simulink model "matlabmodel"  (R2021a)
settings: Solver=VariableStepAuto  StartTime=0.0  StopTime=1  RelTol=1e-3
libraries: spsMosfetLib x8, spsDCVoltageSourceLib x2, spsCurrentMeasurementLib x1, spsSeriesRLCBranchLib x1, spsVoltageMeasurementLib x1, spspowerguiLib x1
settings Model: Creator=welcome  LastModifiedBy=SANJAY

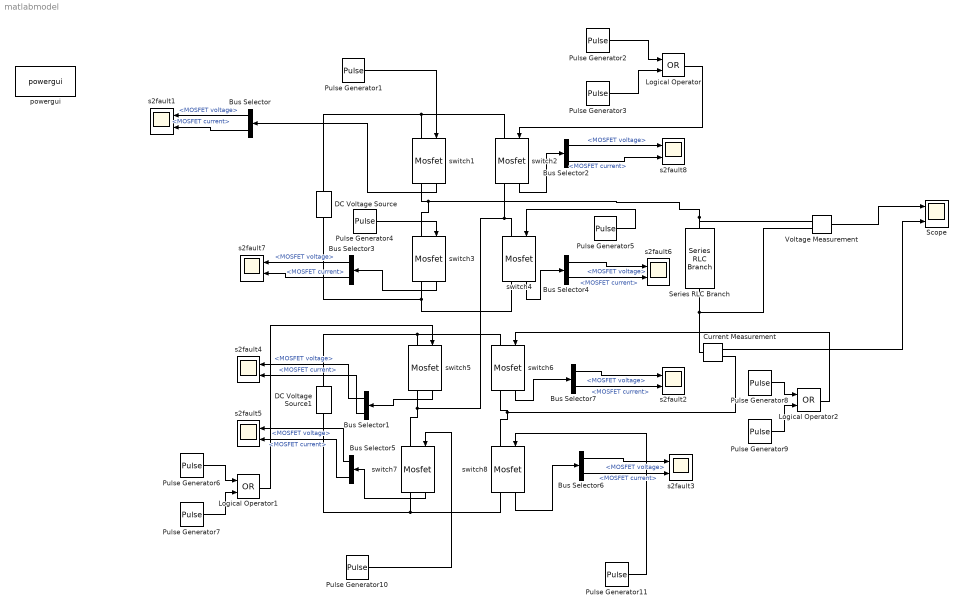
== system matlabmodel ==
  Bus Selector{,1..7} (8 alike) : BusSelector  OutputSignals=MOSFET voltage,MOSFET current
  Current Measurement : spsCurrentMeasurementLib/Current Measurement  PhasorSimulation=off  OutputType=Complex  PSBequivalent=0
  DC Voltage Source : spsDCVoltageSourceLib/DC Voltage Source  Amplitude=100  Measurements=None
  DC Voltage Source1 : spsDCVoltageSourceLib/DC Voltage Source  Amplitude=100  Measurements=None
  Logical Operator : Logic  Operator=OR  AllPortsSameDT=off  OutDataTypeStr=boolean
  Logical Operator1 : Logic  Operator=OR  AllPortsSameDT=off  OutDataTypeStr=boolean
  Logical Operator2 : Logic  Operator=OR  AllPortsSameDT=off  OutDataTypeStr=boolean
  Pulse Generator1 : DiscretePulseGenerator  PulseType=Time based  Period=0.02  PulseWidth=(5/8)*100  PhaseDelay=(0.02/8)*0
  Pulse Generator10 : DiscretePulseGenerator  PulseType=Time based  Period=0.02  PulseWidth=(1/8)*100  PhaseDelay=(0.02/8)*6
  Pulse Generator11 : DiscretePulseGenerator  PulseType=Time based  Period=0.02  PulseWidth=(1/8)*100  PhaseDelay=(0.02/8)*2
  Pulse Generator2 : DiscretePulseGenerator  PulseType=Time based  Period=0.02  PulseWidth=(1/8)*100  PhaseDelay=(0.02/8)*0
  Pulse Generator3 : DiscretePulseGenerator  PulseType=Time based  Period=0.02  PulseWidth=(4/8)*100  PhaseDelay=(0.02/8)*4
  Pulse Generator4 : DiscretePulseGenerator  PulseType=Time based  Period=0.02  PulseWidth=(3/8)*100  PhaseDelay=(0.02/8)*5
  Pulse Generator5 : DiscretePulseGenerator  PulseType=Time based  Period=0.02  PulseWidth=(3/8)*100  PhaseDelay=(0.02/8)*1
  Pulse Generator6 : DiscretePulseGenerator  PulseType=Time based  Period=0.02  PulseWidth=(6/8)*100  PhaseDelay=(0.02/8)*0
  Pulse Generator7 : DiscretePulseGenerator  PulseType=Time based  Period=0.02  PulseWidth=(1/8)*100  PhaseDelay=(0.02/8)*7
  Pulse Generator8 : DiscretePulseGenerator  PulseType=Time based  Period=0.02  PulseWidth=(2/8)*100  PhaseDelay=(0.02/8)*0
  Pulse Generator9 : DiscretePulseGenerator  PulseType=Time based  Period=0.02  PulseWidth=(5/8)*100  PhaseDelay=(0.02/8)*3
  Scope : Scope  NumInputPorts=2
  Series RLC Branch : spsSeriesRLCBranchLib/Series RLC Branch  LConnTagsString=__new0  RConnTagsString=__new0  BranchType=R  Resistance=100  Inductance=1e-3  SetiL0=off  InitialCurrent=0  Capacitance=1e-6  Setx0=off  InitialVoltage=0  Measurements=None
  Voltage Measurement : spsVoltageMeasurementLib/Voltage Measurement  PhasorSimulation=off  OutputType=Complex  PSBequivalent=0
  powergui : spspowerguiLib/powergui  Priority=1  SimulationMode=Continuous  SampleTime=50e-6  frequency=60  Iterations=50  frequencyindice=0  Pbase=100e6  ErrMax=1e-4  UnitsV=kV  UnitsW=MW  buscounter=0  FunctionMessages=off  echomessages=off  EnableUseOfTLC=off  CurrentSourceSwitches=off  DisableSnubberDevices=off  DisableRonSwitches=off  DisableVfSwitches=off  DisplayEquations=off  AutomaticDiscreteSolvers=off  SolverType=Tustin/Backward Euler (TBE)  Interpol=off  ExternalGateDelay=off  methode=off  Ts=100  x0status=blocks  SPID=on  SwTol=0  HookPort=off  NonlinearTolerance=1e-4  nMaxIteration=100  ContinueOnMaxIteration=off  RestoreLinks=warning  ResistiveCurrentMeasurement=off  Frange=[0:2:500]  Ylog=off  Xlog=on  ShowGrid=off  save=off  variable=ZData  structure=0  ZoomFFT=off  StartTime=0.0  cycles=1  DisplayStyle=1  fundamental=60  FreqAxis=off  MaxFrequency=1000  frequencyindicesteady=1  RmsSteady=1  display=off
  s2fault{1..8} (8 alike) : Scope  NumInputPorts=2
  switch{1..8} (8 alike) : spsMosfetLib/Mosfet  Ron=0.1  Lon=0  Rd=0.01  Vfd=0  IC=0  Rs=1e5  Cs=inf  Measurements=on
  wires:
  Pulse Generator2/1 -> Logical Operator/1
  Pulse Generator3/1 -> Logical Operator/2
  Pulse Generator4/1 -> switch3/1
  Pulse Generator5/1 -> switch4/1
  Pulse Generator6/1 -> Logical Operator1/1
  Pulse Generator7/1 -> Logical Operator1/2
  Pulse Generator8/1 -> Logical Operator2/1
  Pulse Generator9/1 -> Logical Operator2/2
  Logical Operator2/1 -> switch6/1
  Logical Operator1/1 -> switch5/1
  Pulse Generator11/1 -> switch8/1
  Pulse Generator10/1 -> switch7/1
  Pulse Generator1/1 -> switch1/1
  switch1/1 -> Bus Selector/1
  Logical Operator/1 -> switch2/1
  Bus Selector/1 -> s2fault1/1  "<MOSFET voltage>"
  switch2/1 -> Bus Selector2/1
  Bus Selector2/1 -> s2fault8/1  "<MOSFET voltage>"
  Bus Selector2/2 -> s2fault8/2  "<MOSFET current>"
  switch3/1 -> Bus Selector3/1
  Bus Selector3/1 -> s2fault7/1  "<MOSFET voltage>"
  Bus Selector3/2 -> s2fault7/2  "<MOSFET current>"
  switch4/1 -> Bus Selector4/1
  Bus Selector4/1 -> s2fault6/1  "<MOSFET voltage>"
  Bus Selector4/2 -> s2fault6/2  "<MOSFET current>"
  switch5/1 -> Bus Selector1/1
  Bus Selector1/1 -> s2fault4/1  "<MOSFET voltage>"
  Bus Selector1/2 -> s2fault4/2  "<MOSFET current>"
  switch7/1 -> Bus Selector5/1
  Bus Selector5/1 -> s2fault5/1  "<MOSFET voltage>"
  Bus Selector5/2 -> s2fault5/2  "<MOSFET current>"
  switch6/1 -> Bus Selector7/1
  Bus Selector7/1 -> s2fault2/1  "<MOSFET voltage>"
  Bus Selector7/2 -> s2fault2/2  "<MOSFET current>"
  switch8/1 -> Bus Selector6/1
  Bus Selector6/1 -> s2fault3/1  "<MOSFET voltage>"
  Bus Selector6/2 -> s2fault3/2  "<MOSFET current>"
  Voltage Measurement/1 -> Scope/1
  Bus Selector/2 -> s2fault1/2  "<MOSFET current>"
  Current Measurement/1 -> Scope/2
  connections:
  switch6/LConn1 -- DC Voltage Source1/RConn1 -- switch5/LConn1
  DC Voltage Source/LConn1 -- switch4/RConn1 -- switch3/RConn1
  switch1/LConn1 -- switch2/LConn1 -- DC Voltage Source/RConn1
  switch4/LConn1 -- switch2/RConn1 -- switch5/RConn1 -- switch7/LConn1
  switch8/LConn1 -- Current Measurement/RConn1 -- switch6/RConn1
  DC Voltage Source1/LConn1 -- switch8/RConn1 -- switch7/RConn1
  Series RLC Branch/LConn1 -- switch3/LConn1 -- switch1/RConn1 -- Voltage Measurement/LConn1
  Series RLC Branch/RConn1 -- Voltage Measurement/LConn2 -- Current Measurement/LConn1
